simulink model "RCAMAircraftsim"  (R2024b)
settings: Solver=VariableStepAuto  StartTime=0.0  StopTime=10.0  RelTol=1e-3
values from neighbouring files (symbols this model uses):
  u1max = 25*pi/180    (= 0.436332312999)    [RCAM_model.m]
  u1min = -25*pi/180    (= -0.436332312999)    [RCAM_model.m]
  u2max = 10*pi/180    (= 0.174532925199)    [RCAM_model.m]
  u2min = -25*pi/180    (= -0.436332312999)    [RCAM_model.m]
  u3max = 30*pi/180    (= 0.523598775598)    [RCAM_model.m]
  u3min = - 30*pi/180    (= -0.523598775598)    [RCAM_model.m]
  u4max = 10*pi/180    (= 0.174532925199)    [RCAM_model.m]
  u5max = 10*pi/180    (= 0.174532925199)    [RCAM_model.m]
  u5min = 0.5*pi/180    (= 0.00872664625997)    [RCAM_model.m]
  UStar = ZStar(10:14)    [Trim.m]    (also in TrimRCAM.m = temp.UStar)
  x0 = [85 ... (first row only)    [sim_initialise.m]
undefined symbols (not defined in the file or in its folder): RCAM_model_new, u14min
settings Model: Creator=satvik_sh  LastModifiedBy=satvik_sh

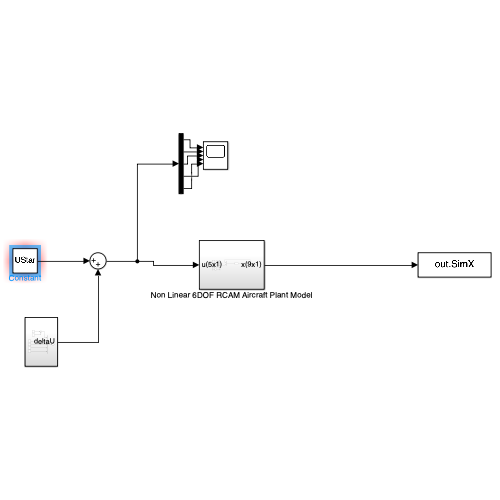
[thumbnail: Simulink's stored preview of the top-level diagram]
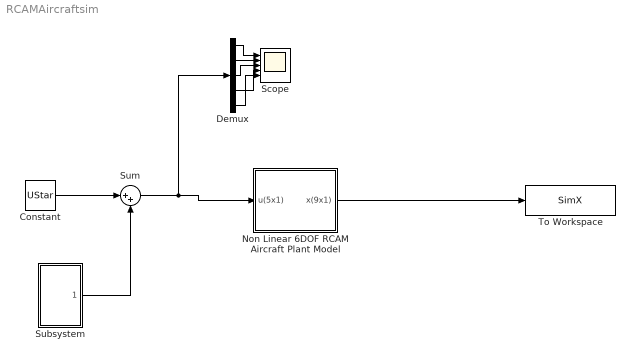
== system RCAMAircraftsim ==
  Constant : Constant  Value=UStar
  Demux : Demux  Outputs=5
  Non Linear 6DOF RCAM Aircraft Plant Model : Subsystem
  Scope : Scope  NumInputPorts=5
  Subsystem : Subsystem
  Sum : Sum  Inputs=|++
  To Workspace : ToWorkspace  VariableName=SimX  SaveFormat=Timeseries  SampleTime=-1
  wires:
  Non Linear 6DOF RCAM Aircraft Plant Model/1(x(9x1)) -> To Workspace/1
  Demux/5 -> Scope/5
  Demux/2 -> Scope/2
  Demux/1 -> Scope/1
  Demux/4 -> Scope/4
  Demux/3 -> Scope/3
  Constant/1 -> Sum/1
  Subsystem/1(deltaU) -> Sum/2
  Sum/1 -> Demux/1, Non Linear 6DOF RCAM Aircraft Plant Model/1(u(5x1))

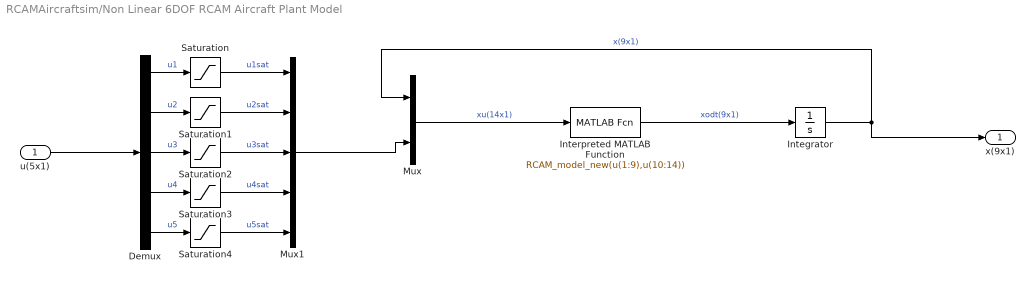
== system RCAMAircraftsim/Non Linear 6DOF RCAM Aircraft Plant Model ==
  u(5x1) : Inport
  Demux : Demux  Outputs=5
  Integrator : Integrator  InitialCondition=x0
  Interpreted MATLAB Function : MATLABFcn  MATLABFcn=RCAM_model_new(u(1:9),u(10:14))
  Mux : Mux  Inputs=2
  Mux1 : Mux  Inputs=5
  Saturation : Saturate  UpperLimit=u1max  LowerLimit=u1min
  Saturation1 : Saturate  UpperLimit=u2max  LowerLimit=u2min
  Saturation2 : Saturate  UpperLimit=u3max  LowerLimit=u3min
  Saturation3 : Saturate  UpperLimit=u4max  LowerLimit=u14min
  Saturation4 : Saturate  UpperLimit=u5max  LowerLimit=u5min
  x(9x1) : Outport
  wires:
  Interpreted MATLAB Function/1 -> Integrator/1  "xodt(9x1)"
  Mux/1 -> Interpreted MATLAB Function/1  "xu(14x1)"
  Integrator/1 -> x(9x1)/1, Mux/1  "x(9x1)"
  u(5x1)/1 -> Demux/1
  Demux/1 -> Saturation/1  "u1"
  Demux/2 -> Saturation1/1  "u2"
  Demux/3 -> Saturation2/1  "u3"
  Demux/4 -> Saturation3/1  "u4"
  Demux/5 -> Saturation4/1  "u5"
  Saturation/1 -> Mux1/1  "u1sat"
  Saturation1/1 -> Mux1/2  "u2sat"
  Saturation2/1 -> Mux1/3  "u3sat"
  Saturation3/1 -> Mux1/4  "u4sat"
  Saturation4/1 -> Mux1/5  "u5sat"
  Mux1/1 -> Mux/2

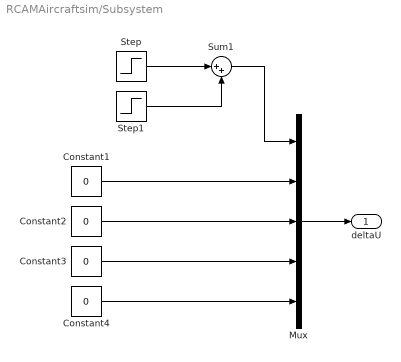
== system RCAMAircraftsim/Subsystem ==
  Constant{1..4} (4 alike) : Constant  Value=0
  Mux : Mux  Inputs=5
  Step : Step  Time=5  After=5*pi/180  SampleTime=0
  Step1 : Step  Time=6  After=-5*pi/180  SampleTime=0
  Sum1 : Sum  Inputs=|++
  deltaU : Outport
  wires:
  Constant3/1 -> Mux/4
  Step1/1 -> Sum1/2
  Constant4/1 -> Mux/5
  Step/1 -> Sum1/1
  Constant1/1 -> Mux/2
  Sum1/1 -> Mux/1
  Mux/1 -> deltaU/1
  Constant2/1 -> Mux/3
